simulink model "Blind_Spot_Monitoring"  (R2025a)
settings: Solver=FixedStepAuto  StartTime=0.0  StopTime=30  RelTol=1e-3
libraries: SignalEditorBlockLib x1
settings Model: Creator=Rudransh  LastModifiedBy=Rudransh
settings OptimizationCC: DefaultParameterBehavior=Inlined  EnhancedBackFolding=on  PassReuseOutputArgsAs=Individual arguments  ZeroExternalMemoryAtStartup=off  ZeroInternalMemoryAtStartup=off  OptimizeBlockOrder=speed  DifferentSizesBufferReuse=on  OptimizationCustomize=off  EfficientTunableParamExpr=on
settings DebuggingCC: ParameterTunabilityLossMsg=error
settings SFSimCC: MATLABDynamicMemAlloc=off
settings RTWCC: SystemTargetFile=autosar.tlc  GenCodeOnly=on  TemplateMakefile=ert_default_tmf  DataTypeReplacement=CDataTypesFixedWidth  Description=AUTOSAR
settings CodeAppCC: ForceParamTrailComments=on  IgnoreCustomStorageClasses=off  OperatorAnnotations=on  SimulinkDataObjDesc=on  SFDataObjDesc=on  InsertBlockDesc=on
settings STFCustomTargetCC: SystemTargetFile=autosar.tlc  TargetLangStandard=C99 (ISO)  MultiwordLength=256.0  DynamicStringBufferSize=256.0  ParMdlRefBuildCompliant=on  CompOptLevelCompliant=on  IncludeMdlTerminateFcn=off  CombineOutputUpdateFcns=on  SuppressErrorStatus=on  ERTCustomFileBanners=on  SupportNonFinite=off  SupportComplex=off  SupportContinuousTime=off  SupportNonInlinedSFcns=off  RemoveResetFunc=on  MATLABClassNameForMDSCustomization=Simulink.SoftwareTarget.ERTCustomization  AutosarCompliant=on  GRTInterface=off  UseToolchainInfoCompliant=on  LookupTableObjectStructAxisOrder=2,1,3,4,...  LUTObjectStructOrderEvenSpacing=Size,Table,Breakpoints  AutosarMatrixIOAsArray=off  AutosarSchemaVersion=R23-11  DisableAUTOSARRoutinesHostLibrary=off  AutosarCompilerAbstraction=off  AutosarMaxShortNameLength=128.0
settings ERTTargetCC: ExtModeTransport=0.0  ExtModeStaticAlloc=off  ExtModeMexFile=ext_comm  ExtModeIntrfLevel=Level1  ERTCustomFileTemplate=example_file_process.tlc  BooleanTrueId=TRUE  BooleanFalseId=FALSE  TargetLangStandard=C99 (ISO)  ConcurrentExecutionCompliant=off  IncludeMdlTerminateFcn=off  SuppressErrorStatus=on  SupportNonFinite=off  SupportComplex=off  ModelStepFunctionPrototypeControlCompliant=off  CPPClassGenCompliant=off  AutosarCompliant=on  LookupTableObjectStructAxisOrder=2,1,3,4,...  LUTObjectStructOrderEvenSpacing=Size,Table,Breakpoints

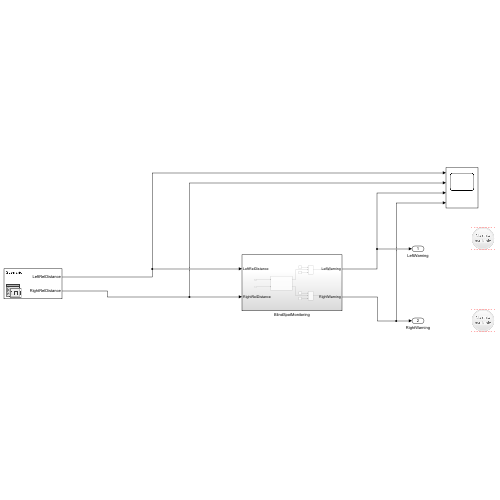
[thumbnail: Simulink's stored preview of the top-level diagram]
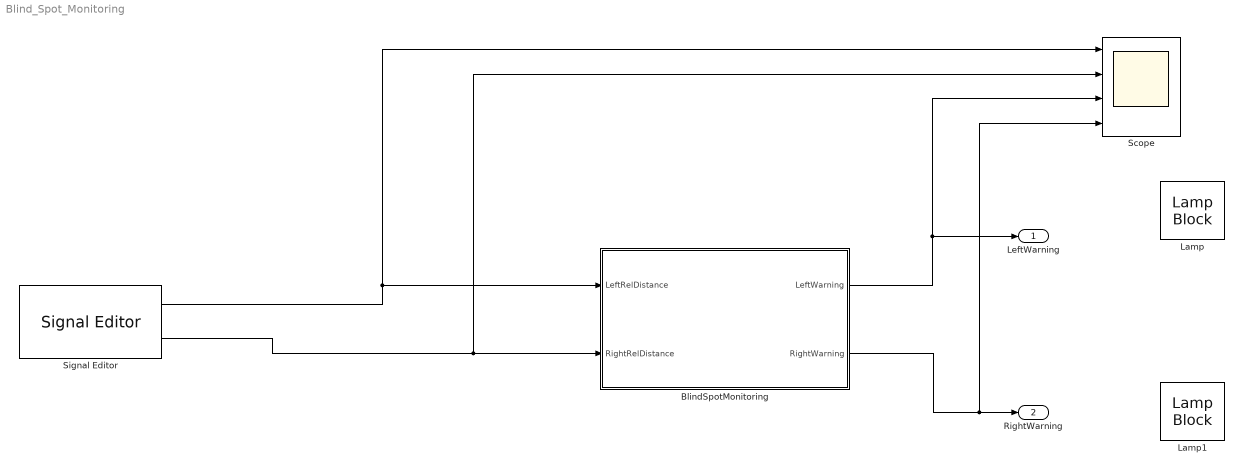
== system Blind_Spot_Monitoring ==
  BlindSpotMonitoring : Subsystem
  Lamp : LampBlock  LabelPosition=Hide  DefaultColor=[192.0, 192.0, 192.0]
  Lamp1 : LampBlock  LabelPosition=Hide  DefaultColor=[192.0, 192.0, 192.0]
  Scope : Scope  NumInputPorts=4
      settings: ActiveDisplayString=4  Title=RightWarning  ActiveDisplayYMinimum=0  ActiveDisplayYMaximum=1
  Signal Editor : SignalEditorBlockLib/Signal Editor  FileName=C:\Projects_ESD\AUTOSAR_CARSYSTEM\ADAS\Blind_Spot_Monitoring\Scenario\ScenarioBSM.mat  ActiveScenario=Scenario  ActiveSignal=LeftRelDistance  IsBus=off  OutputBusObjectStr=Bus: BusObject  SampleTime=0  ZeroCross=off  OutputAfterFinalValue=Setting to zero  Unit=inherit  PreserveSignalName=on  ApplySigPropsToAllScenarios=on  ApplySigPropsToAllSignals=off  SignalPropertySource=Dialog parameters
  LeftWarning : Outport
  RightWarning : Outport  Port=2
  wires:
  BlindSpotMonitoring/1(LeftWarning) -> Scope/3, LeftWarning/1
  BlindSpotMonitoring/2(RightWarning) -> Scope/4, RightWarning/1
  Signal Editor/1 -> Scope/1, BlindSpotMonitoring/1(LeftRelDistance)
  Signal Editor/2 -> Scope/2, BlindSpotMonitoring/2(RightRelDistance)

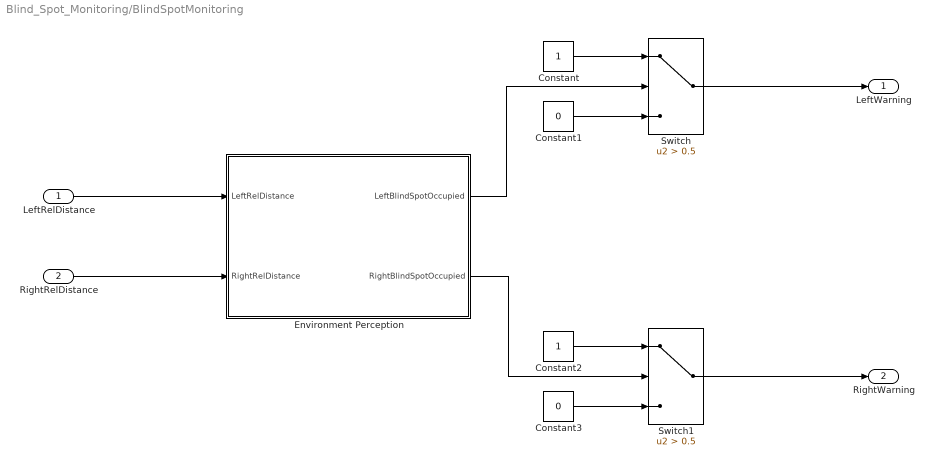
== system Blind_Spot_Monitoring/BlindSpotMonitoring ==
  LeftRelDistance : Inport
  RightRelDistance : Inport  Port=2
  Constant : Constant
  Constant1 : Constant  Value=0
  Constant2 : Constant
  Constant3 : Constant  Value=0
  Environment Perception : Subsystem
  Switch : Switch  Criteria=u2 > Threshold  Threshold=0.5  SaturateOnIntegerOverflow=off  InputSameDT=off
  Switch1 : Switch  Criteria=u2 > Threshold  Threshold=0.5  SaturateOnIntegerOverflow=off  InputSameDT=off
  LeftWarning : Outport
  RightWarning : Outport  Port=2
  wires:
  Constant3/1 -> Switch1/3
  Environment Perception/1(LeftBlindSpotOccupied) -> Switch/2
  RightRelDistance/1 -> Environment Perception/2(RightRelDistance)
  Switch1/1 -> RightWarning/1
  Constant/1 -> Switch/1
  LeftRelDistance/1 -> Environment Perception/1(LeftRelDistance)
  Constant2/1 -> Switch1/1
  Constant1/1 -> Switch/3
  Switch/1 -> LeftWarning/1
  Environment Perception/2(RightBlindSpotOccupied) -> Switch1/2

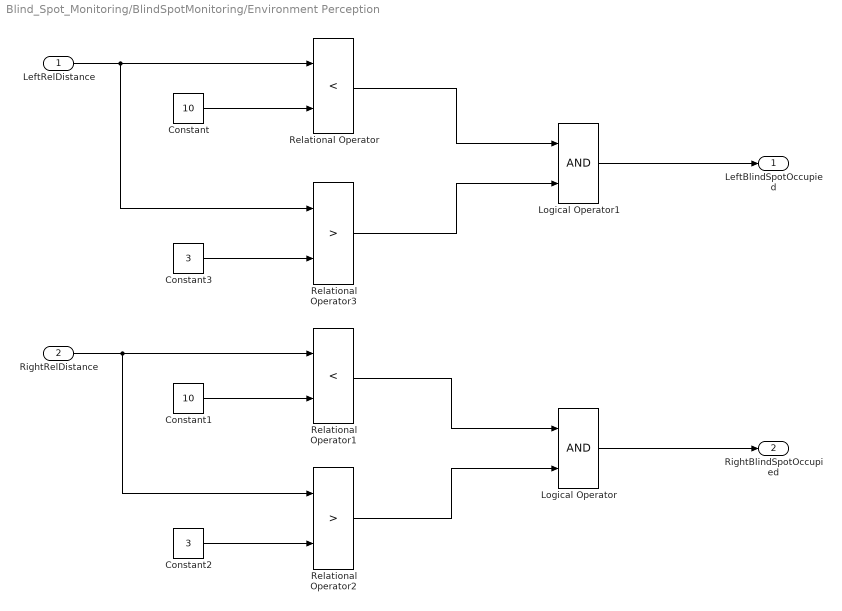
== system Blind_Spot_Monitoring/BlindSpotMonitoring/Environment Perception ==
  LeftRelDistance : Inport
  RightRelDistance : Inport  Port=2
  Constant : Constant  Value=10
  Constant1 : Constant  Value=10
  Constant2 : Constant  Value=3
  Constant3 : Constant  Value=3
  Logical Operator : Logic  AllPortsSameDT=off  OutDataTypeStr=boolean
  Logical Operator1 : Logic  AllPortsSameDT=off  OutDataTypeStr=boolean
  Relational Operator : RelationalOperator  Operator=<  OutDataTypeStr=boolean  RndMeth=Simplest  InputSameDT=off
  Relational Operator1 : RelationalOperator  Operator=<  OutDataTypeStr=boolean  RndMeth=Simplest  InputSameDT=off
  Relational Operator2 : RelationalOperator  Operator=>  OutDataTypeStr=boolean  RndMeth=Simplest  InputSameDT=off
  Relational Operator3 : RelationalOperator  Operator=>  OutDataTypeStr=boolean  RndMeth=Simplest  InputSameDT=off
  LeftBlindSpotOccupied : Outport
  RightBlindSpotOccupied : Outport  Port=2
  wires:
  Constant2/1 -> Relational Operator2/2
  RightRelDistance/1 -> Relational Operator2/1, Relational Operator1/1
  Constant1/1 -> Relational Operator1/2
  Relational Operator2/1 -> Logical Operator/2
  LeftRelDistance/1 -> Relational Operator3/1, Relational Operator/1
  Logical Operator1/1 -> LeftBlindSpotOccupied/1
  Relational Operator1/1 -> Logical Operator/1
  Relational Operator/1 -> Logical Operator1/1
  Constant/1 -> Relational Operator/2
  Logical Operator/1 -> RightBlindSpotOccupied/1
  Constant3/1 -> Relational Operator3/2
  Relational Operator3/1 -> Logical Operator1/2
